simulink model "Hinf"  (R2022b)
settings: Solver=VariableStepAuto  StartTime=0.0  StopTime=10.0  RelTol=1e-3
values from neighbouring files (symbols this model uses):
  dem_alpha = [1 87 0]    [Data.mat]
  dem_nz = [1 745.7079 0]    [Data.mat]
  dem_q = [1 11493 147030 251760 0]    [Data.mat]
  num_alpha = [981.3252 6287.3 1497.7]    [Data.mat]
  num_nz = [-0.5655 -111.5642 -1509.3]    [Data.mat]
  num_q = [-0.0368 -6.05 -119.3225 -3899.3 -28044]    [Data.mat]
libraries: simulink x2
settings Model: Creator=KIWI  LastModifiedBy=KIWI

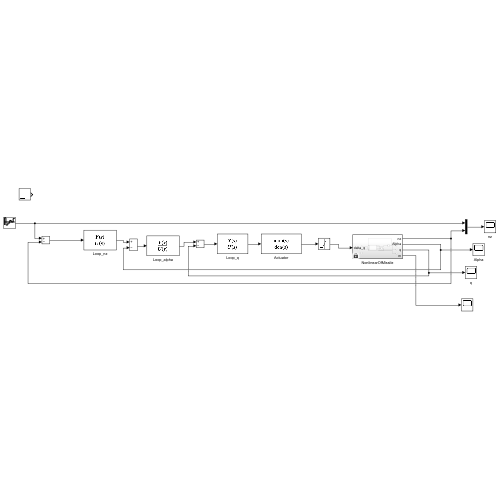
[thumbnail: Simulink's stored preview of the top-level diagram]
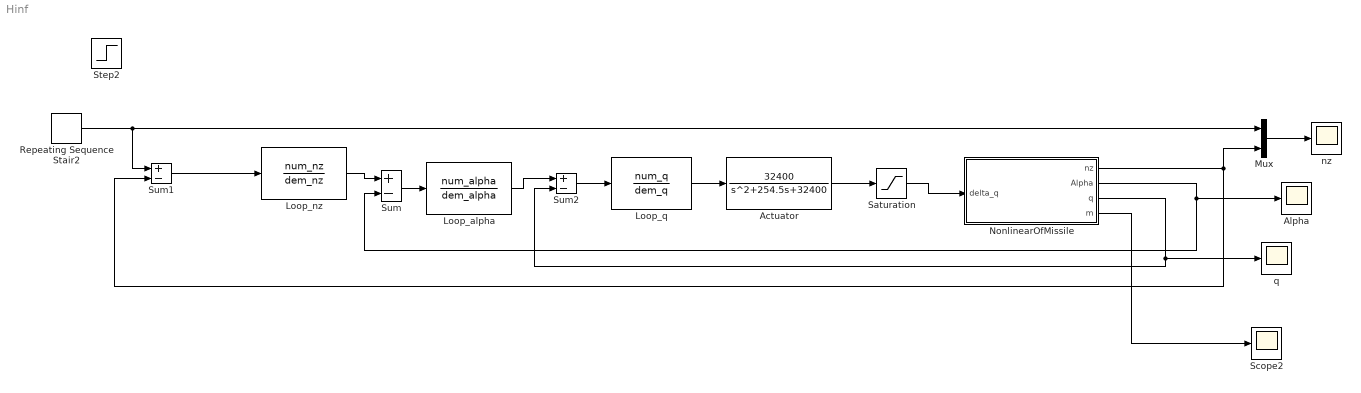
== system Hinf ==
  Actuator : TransferFcn  Numerator=32400  Denominator=[1 254.5 32400]
  Alpha : Scope
  Loop_alpha : TransferFcn  Numerator=num_alpha  Denominator=dem_alpha
  Loop_nz : TransferFcn  Numerator=num_nz  Denominator=dem_nz
  Loop_q : TransferFcn  Numerator=num_q  Denominator=dem_q
  Mux : Mux  Inputs=2
  NonlinearOfMissile : Subsystem
      settings: PermitHierarchicalResolution=None  MinAlgLoopOccurrences=on
  Repeating Sequence Stair2 : simulink/Sources/Repeating Sequence Stair  OutValues=[50 -40 -15 15 -1 40]  tsamp=2  OutMin=[]  OutMax=[]  OutDataTypeStr=double  OutputDataTypeScalingMode=double  OutDataType=fixdt(0,8)  ConRadixGroup=Best Precision: Vector-wise  OutScaling=2^-12
  Saturation : Saturate  UpperLimit=30  LowerLimit=-30
  Scope2 : Scope
  Step2 : Step  Time=0  Before=10  After=10  SampleTime=0
  Sum : Sum  Inputs=+-
  Sum1 : Sum  Inputs=+-
  Sum2 : Sum  Inputs=+-
  nz : Scope
  q : Scope
  wires:
  Repeating Sequence Stair2/1 -> Mux/1, Sum1/1
  Sum1/1 -> Loop_nz/1
  NonlinearOfMissile/1(nz) -> Mux/2, Sum1/2
  Loop_nz/1 -> Sum/1
  Loop_alpha/1 -> Sum2/1
  Loop_q/1 -> Actuator/1
  NonlinearOfMissile/3(q) -> Sum2/2, q/1
  NonlinearOfMissile/2(Alpha) -> Sum/2, Alpha/1
  NonlinearOfMissile/4(m) -> Scope2/1
  Actuator/1 -> Saturation/1
  Mux/1 -> nz/1
  Sum/1 -> Loop_alpha/1
  Sum2/1 -> Loop_q/1
  Saturation/1 -> NonlinearOfMissile/1(delta_q)

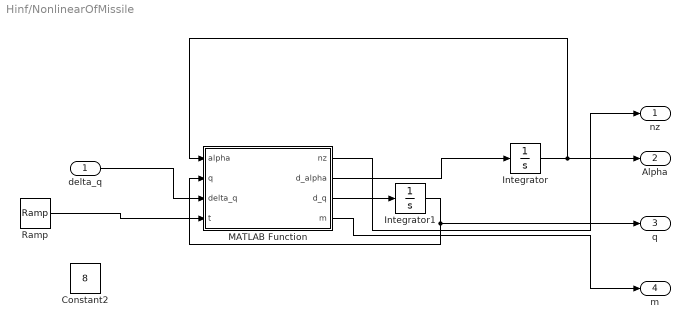
== system Hinf/NonlinearOfMissile ==
  delta_q : Inport
  Constant2 : Constant  Value=8
  Integrator : Integrator
  Integrator1 : Integrator
  MATLAB Function : MATLAB Function  TreatAsAtomicUnit=on
  Ramp : simulink/Sources/Ramp  slope=1  start=0  InitialOutput=0
  nz : Outport
  Alpha : Outport  Port=2
  q : Outport  Port=3
  m : Outport  Port=4
  wires:
  MATLAB Function/3(d_q) -> Integrator1/1
  Integrator1/1 -> MATLAB Function/2(q), q/1
  MATLAB Function/2(d_alpha) -> Integrator/1
  MATLAB Function/4(m) -> m/1
  Integrator/1 -> MATLAB Function/1(alpha), Alpha/1
  delta_q/1 -> MATLAB Function/3(delta_q)
  MATLAB Function/1(nz) -> nz/1
  Ramp/1 -> MATLAB Function/4(t)

== matlab function Hinf/NonlinearOfMissile/MATLAB Function ==
  data: nz output; d_alpha output; d_q output; alpha input; q input; delta_q input; t input; m output
function [nz, d_alpha, d_q, m] = myMissile(alpha, q, delta_q, t)
%Init missile data
h = 6000; % Do cao bay cua TL
g = 9.8;
Makha = 316; % Toc do am thanh o do cao 6000m 
Vm = 2.5*Makha; % Toc do TL
ro_0 = 0.125;   % Mat do khong khi o dieu kien binh thuong
ro = ro_0*(1-h/44300)*4.256;    % ???
ro = 0.66;  % kg/m3, do cao h = 6000m https://www.engineeringtoolbox.com/international-standard-atmosphere-d_985.html
qm = ro*Vm^2/2; % Ap suat dong, N/m2

Sref = 3.0828; % Table C.1
d = 0.1981; % Table C.1
Se = pi*d^2/4; %7.947*10^-2;% Table C.1
L_missile = 2.972; % m. Table C.1
L_momentcenter = 1.4562; % m  Table C.2
L_masscenter_launch = 1.4858;
L_masscenter_endboots = 1.4362;
L_masscenter_burnout = 1.2877;

m1 = 101.3; % 87.27 kg (burn out);
Iy_b1 = 33.2;  % (m = 101.3kg) Table C.2:  35.6 -> 129.2kg; 32 -> 87.27kg
s_ngang1 = (L_masscenter_endboots - L_momentcenter)/d;    % -0.25

m2 = 87.27;
Iy_b2 = 32;
s_ngang2 = (L_masscenter_burnout - L_momentcenter)/d;   % -0.85 Table 4.2

t_bourning = 8; % Burning time
d_m = (m1 - m2)/t_bourning;
d_Iy = (Iy_b1-Iy_b2)/t_bourning;
d_s_ngang = (s_ngang1 - s_ngang2)/t_bourning;
if t <= t_bourning
    m = m1 - t*d_m;
    Iy_b = Iy_b1 - t * d_Iy;
    s_ngang = s_ngang1 - t*d_s_ngang;
else
    m = m2;
    Iy_b = Iy_b2;
    s_ngang = s_ngang2;
end
% Bieu thu tinh cac he so
Ca_0 = 4.362*10^-1;% Table E.5 page 211
deltaCa_b = 1.062*10^-1;% Table E.5 page 211

T = 3400; % N. Table C.2
Ct = T/(qm*Sref);
Ct = 1.2;   % Table 4.4

Cn_alphacube = -1.131*10^-5;% Table E.2 page 207
Cn_alpha = 2.020*10^-1;% Table E.2 page 207
Cn_alpha_absalpha = 1.110*10^-2;
Cn_alphadot = -2.781*10^-2; % Table E.2
Cn_q = 5.734*10^-1;% Table E.2 page 207

Ca_alpha = 3.886*10^-3; % Table E.5 page 211
Ca_alphasqua = -7.642*10^-5; % % Table E.5 page 211
Ca_alphacube = 2.111*10^-6; % Table E.5 page 211
Ca_deltaq = -2.282*10^-2; % Table E.5 page 211
Ca_alpha_deltaq = 1.904*10^-3; % Table E.5 page 211
Ca_alphasqua_deltaq = -2.708*10^-5; % Table E.5 page 211
Cn_deltaq = 6.961*10^-2; % Table E.2 page 207
Cn_alpha_deltaq = 4.066*10^-4; % Table E.2 page 208

Cm_alpha = 1.373*10^-1; % Table E.3 page 208
Cm_alpha_absalpha = -1.020*10^-2; % Table E.3 page 208
Cm_alphacube = -6.864*10^-5; % Table E.3 page 208
Cm_q = -18.560; % Table E.3 page 209

Cm_0alpha_deltaq = -5.014*10^-1;%Table E.3
Cm_1alpha_deltaq = 3.520*10^-3;%Table E.3
Cm_2alpha_deltaq = 1.384*10^-4; %Table E.3
Cm_3alpha_deltaq = -1.705*10^-5; %Table E.3
Cm_4alpha_deltaq = 1.916*10^-7; %Table E.3
%Cm_deltaq = Cm_0_alphadeltaq; % +/- ...  Equation 3.51 page 66

%alpha = 20; % degree
%delta_q = 10; % degree

if alpha >= 0
    Cm_alpha_deltaq = Cm_0alpha_deltaq + Cm_1alpha_deltaq*alpha + Cm_2alpha_deltaq*alpha^2 ...
    + Cm_3alpha_deltaq*alpha^3 + Cm_4alpha_deltaq*alpha^4;
else
    Cm_alpha_deltaq = 2*Cm_0alpha_deltaq - Cm_1alpha_deltaq*abs(alpha) - Cm_2alpha_deltaq*abs((alpha))^2 ...
    - Cm_3alpha_deltaq*(abs(alpha))^3 - Cm_4alpha_deltaq*(abs(alpha))^4;
end

if alpha == 0
    mysinc = 1;
else
    mysinc = sind(alpha)/alpha;
end

D_alphadot = 1 + qm*Sref*cosd(alpha)*d*Cn_alphadot/(2*m*Vm^2);
a11 = qm*Sref*(sind(alpha)*(Ca_alpha + Ca_alphasqua*abs(alpha) + Ca_alphacube*alpha^2)*sign(alpha)...
    + mysinc*(Ca_0 + deltaCa_b - Ct) - ...
    cosd(alpha)*(Cn_alpha + Cn_alpha_absalpha*abs(alpha)...
    + Cn_alphacube*alpha^2)) / (m*Vm*D_alphadot);
a12 = (1 - qm*Sref*d*cosd(alpha)*Cn_q/(2*m*Vm^2)) / D_alphadot;
a21 = qm*Sref*d*(Cm_alpha + Cm_alpha_absalpha*abs(alpha)+ Cm_alphacube*alpha^2 + ...
    s_ngang*(Cn_alpha + Cn_alpha_absalpha*abs(alpha) + Cn_alphacube*alpha^2)) / Iy_b;
a22 = (qm*Sref*d^2)*(Cm_q + s_ngang*Cn_q) / (2*Vm*Iy_b);
b11 = qm*Sref*( (sind(alpha)*Ca_deltaq*sign(delta_q) - cosd(alpha)*Cn_deltaq) + ...
    alpha*(sind(alpha)*Ca_alpha_deltaq - cosd(alpha)*Cn_alpha_deltaq) + ...
    sind(alpha)*Ca_alphasqua_deltaq*alpha^2) / (m*Vm*D_alphadot);
b21 = qm*Sref*d*(Cm_alpha_deltaq + s_ngang*(Cn_deltaq + alpha*Cn_alpha_deltaq)) / Iy_b;

% Normal acceleration
c11 = -qm*Se*(Cn_alpha + Cn_alpha_absalpha*abs(alpha)+Cn_alphacube*alpha^2+Cn_alphadot*d*a11/(2*Vm))/m;
%c11 = c11/g;
c12 = -qm*Se*d*(Cn_q + Cn_alphadot*a12)/(2*m*Vm);
%c12 = c12/g;
d11 = -qm*Se*(Cn_deltaq + Cn_alpha_deltaq*alpha + Cn_alphadot*d*b11/(2*Vm))/m;
%d11 = d11/g;

% State space equations
d_alpha = a11*alpha + a12*q + b11*delta_q;
d_q     = a21*alpha + a22*q + b21*delta_q;

nz = c11*alpha + c12*q + d11*delta_q;
%q  = 0*alpha   + 1*q   + 0*delta_q;
nz = nz/g;
